simulink model "Project4_MODEL_FINAL"  (R2024b)
settings: Solver=ode45  StartTime=0.0  StopTime=600  RelTol=1e-3
values from neighbouring files (symbols this model uses):
  x_center = [x1 x2_adjusted transition_x x3_adjusted x4]    [Project4_FINAL_Script.m]
  y_center = [y1 y2_adjusted transition_y y3_adjusted y4]    [Project4_FINAL_Script.m]
undefined symbols (not defined in the file or in its folder): BattData, carData, motorData
libraries: slpidlib x1
settings Model: Creator=saman  LastModifiedBy=gabes
settings RTWCC: GPUComputeCapability=3.5

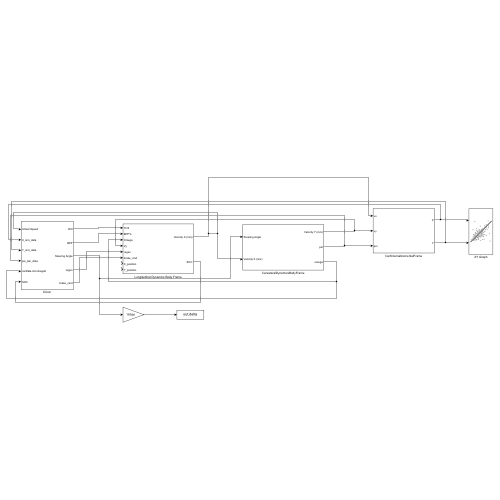
[thumbnail: Simulink's stored preview of the top-level diagram]
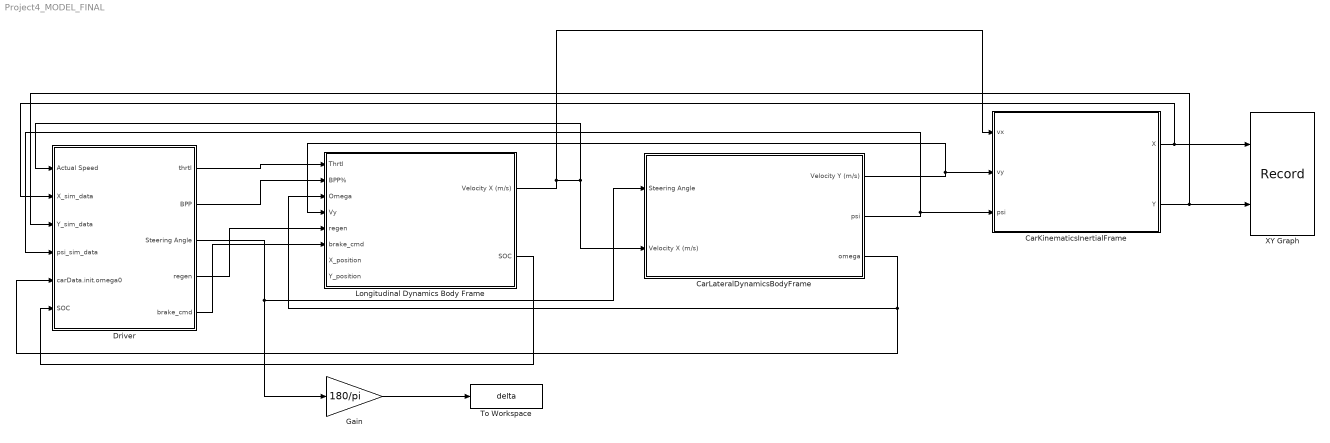
== system Project4_MODEL_FINAL ==
  CarKinematicsInertialFrame : Subsystem
  CarLateralDynamicsBodyFrame : Subsystem
  "Driver " : Subsystem
  Gain : Gain  Gain=180/pi
  Longitudinal Dynamics Body Frame : Subsystem
  To Workspace : ToWorkspace  VariableName=delta  SaveFormat=Timeseries  SampleTime=-1
  XY Graph : Record  FileSettingsInternal="{\"entries\":[{\"content\":{\"excelSettings\":{\"content\":{},\"type\":\"Streamout.ExcelSettings\"}},\"type\":\"Streamout.FileSettingStorage\",\"uuid\":\"\"}],\"packageUris\":[\"http:\\/\\/schema.mathworks.com\\/mf0\\/streamout_blocks\\/R2020a\"],\"version\":\"1.0\"}"  Layout=[1 1]  SignalsInternal="{\"entries\":[{\"content\":{\"signals\":[{\"content\":{\"blockPath\":[],\"dimensions\":[1],\"domain\":\"\",\"lineColor\":\"#a2142f\",\"plots\":[ 1 ],\"port\":1,\"sid\":[\"\"],\"signalID\":1,\"signalName\":\"CarKinematicsInertialFrame:1\"},\"type\":\"RecordBlkView.Signal\",\"uuid\":\"\"},{\"content\":{\"blockPath\":[],\"dimensions\":[1],\"domain\":\"\",\"lineColor\":\"#139fff\",\"plots\":[ 1 ],\"port\":2,\"sid\":[\"\"],\"signalID\":2,\"signalName\":\"CarKinematicsInertialFrame:2\"},\"type\":\"RecordBlkView.Signal\",\"uuid\":\"\"}]},\"type\":\"RecordBlkView.InputSignals\",\"uuid\":\"\"}],\"packageUris\":[\"http:\\/\\/schema.mathworks.com\\/mf0\\/streamout_blocks\\/R2020a\"],\"version\":\"1.0\"}"  VisualizationBindings="{\"xyplotplugin\":{\"info\":[{\"series\":[{\"bindingParametersList\":[{\"parameter\":\"X-Axis\",\"signalID\":1,\"signalName\":\"CarKinematicsInertialFrame:1\"},{\"parameter\":\"Y-Axis\",\"signalID\":2,\"signalName\":\"CarKinematicsInertialFrame:2\"}],\"seriesID\":0}],\"subplotID\":1}]}}"  CompatibilityTag=XY  st=-1
  wires:
  CarLateralDynamicsBodyFrame/2(psi) -> "Driver "/4(psi_sim_data), CarKinematicsInertialFrame/3(psi)
  CarKinematicsInertialFrame/2(Y) -> "Driver "/3(Y_sim_data), XY Graph/2
  CarKinematicsInertialFrame/1(X) -> XY Graph/1, "Driver "/2(X_sim_data)
  CarLateralDynamicsBodyFrame/1(Velocity Y (m/s)) -> Longitudinal Dynamics Body Frame/4(Vy), CarKinematicsInertialFrame/2(vy)
  "Driver "/1(thrtl) -> Longitudinal Dynamics Body Frame/1(Thrtl)
  "Driver "/2(BPP) -> Longitudinal Dynamics Body Frame/2(BPP%)
  Longitudinal Dynamics Body Frame/1(Velocity X (m/s)) -> CarKinematicsInertialFrame/1(vx), "Driver "/1(Actual Speed), CarLateralDynamicsBodyFrame/2(Velocity X (m/s))
  Longitudinal Dynamics Body Frame/2(SOC) -> "Driver "/6(SOC)
  CarLateralDynamicsBodyFrame/3(omega) -> Longitudinal Dynamics Body Frame/3(Omega), "Driver "/5(carData.init.omega0)
  "Driver "/3(Steering Angle) -> Gain/1, CarLateralDynamicsBodyFrame/1(Steering Angle)
  Gain/1 -> To Workspace/1
  "Driver "/4(regen) -> Longitudinal Dynamics Body Frame/5(regen)
  "Driver "/5(brake_cmd) -> Longitudinal Dynamics Body Frame/6(brake_cmd)

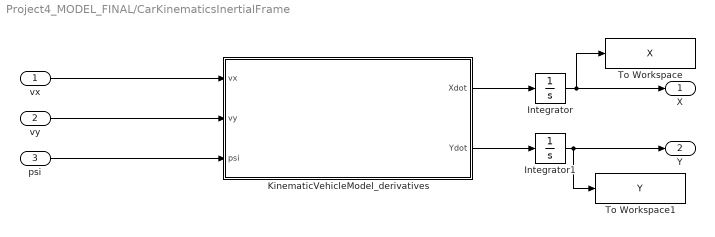
== system Project4_MODEL_FINAL/CarKinematicsInertialFrame ==
  vx : Inport
  vy : Inport  Port=2
  psi : Inport  Port=3
  Integrator : Integrator  InitialCondition=carData.init.x0
  Integrator1 : Integrator  InitialCondition=carData.init.y0
  KinematicVehicleModel_derivatives : MATLAB Function  TreatAsAtomicUnit=on  mask{obj=carData}
      mask prompts: obj "obj structure"
  To Workspace : ToWorkspace  VariableName=X  SaveFormat=Timeseries  SampleTime=-1
  To Workspace1 : ToWorkspace  VariableName=Y  SaveFormat=Timeseries  SampleTime=-1
  X : Outport
  Y : Outport  Port=2
  wires:
  KinematicVehicleModel_derivatives/1(Xdot) -> Integrator/1
  KinematicVehicleModel_derivatives/2(Ydot) -> Integrator1/1
  Integrator/1 -> To Workspace/1, X/1
  Integrator1/1 -> To Workspace1/1, Y/1
  vx/1 -> KinematicVehicleModel_derivatives/1(vx)
  vy/1 -> KinematicVehicleModel_derivatives/2(vy)
  psi/1 -> KinematicVehicleModel_derivatives/3(psi)

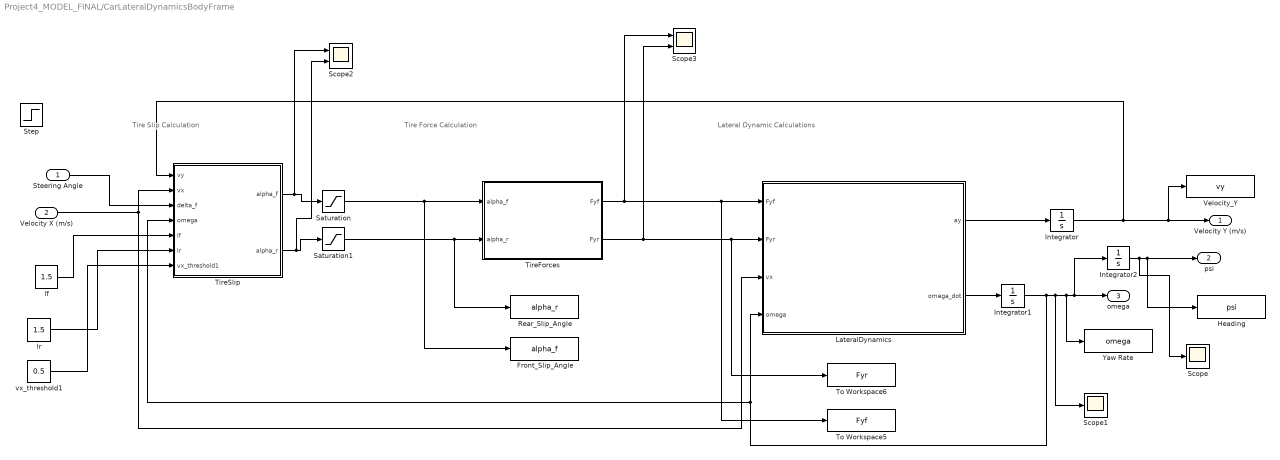
== system Project4_MODEL_FINAL/CarLateralDynamicsBodyFrame ==
  note: Tire Slip Calculation
  note: Tire Force Calculation
  note: Lateral Dynamic Calculations
  Steering Angle : Inport
  Velocity X (m/s) : Inport  Port=2
  Front_Slip_Angle : ToWorkspace  VariableName=alpha_f  SaveFormat=Timeseries  SampleTime=-1
  Heading : ToWorkspace  VariableName=psi  SaveFormat=Timeseries  SampleTime=-1
  Integrator : Integrator  InitialCondition=carData.init.vy0
  Integrator1 : Integrator  InitialCondition=carData.init.omega0
  Integrator2 : Integrator  InitialCondition=carData.init.psi0
  LateralDynamics : MATLAB Function  TreatAsAtomicUnit=on  mask{obj=carData}
      mask prompts: obj "obj structure"
  Rear_Slip_Angle : ToWorkspace  VariableName=alpha_r  SaveFormat=Timeseries  SampleTime=-1
  Saturation : Saturate  UpperLimit=carData.maxAlpha  LowerLimit=-carData.maxAlpha
  Saturation1 : Saturate  UpperLimit=carData.maxAlpha  LowerLimit=-carData.maxAlpha
  Scope : Scope
  Scope1 : Scope
  Scope2 : Scope  NumInputPorts=2
  Scope3 : Scope  NumInputPorts=2
  Step : Step  Time=180  SampleTime=10
  TireForces : MATLAB Function  TreatAsAtomicUnit=on  mask{obj=carData}
      mask prompts: obj "obj structure"
  TireSlip : MATLAB Function  TreatAsAtomicUnit=on  mask{obj=carData}
      mask prompts: obj "obj structure"
  To Workspace5 : ToWorkspace  VariableName=Fyf  SaveFormat=Timeseries  SampleTime=-1
  To Workspace6 : ToWorkspace  VariableName=Fyr  SaveFormat=Timeseries  SampleTime=-1
  Velocity_Y : ToWorkspace  VariableName=vy  SaveFormat=Timeseries  SampleTime=-1
  Yaw Rate : ToWorkspace  VariableName=omega  SaveFormat=Timeseries  SampleTime=-1
  lf : Constant  Value=1.5
  lr : Constant  Value=1.5
  vx_threshold1 : Constant  Value=0.5
  Velocity Y (m/s) : Outport
  psi : Outport  Port=2
  omega : Outport  Port=3
  wires:
  LateralDynamics/1(ay) -> Integrator/1
  Integrator/1 -> Velocity Y (m/s)/1, Velocity_Y/1, TireSlip/1(vy)
  LateralDynamics/2(omega_dot) -> Integrator1/1
  Integrator1/1 -> Scope1/1, Integrator2/1, omega/1, Yaw Rate/1, LateralDynamics/4(omega), TireSlip/4(omega)
  TireSlip/1(alpha_f) -> Scope2/1, Saturation/1
  TireSlip/2(alpha_r) -> Scope2/2, Saturation1/1
  TireForces/2(Fyr) -> Scope3/2, LateralDynamics/2(Fyr), To Workspace6/1
  Saturation/1 -> TireForces/1(alpha_f), Front_Slip_Angle/1
  Saturation1/1 -> TireForces/2(alpha_r), Rear_Slip_Angle/1
  Velocity X (m/s)/1 -> TireSlip/2(vx), LateralDynamics/3(vx)
  Integrator2/1 -> Scope/1, Heading/1, psi/1
  vx_threshold1/1 -> TireSlip/7(vx_threshold1)
  lf/1 -> TireSlip/5(lf)
  lr/1 -> TireSlip/6(lr)
  TireForces/1(Fyf) -> Scope3/1, To Workspace5/1, LateralDynamics/1(Fyf)
  Steering Angle/1 -> TireSlip/3(delta_f)

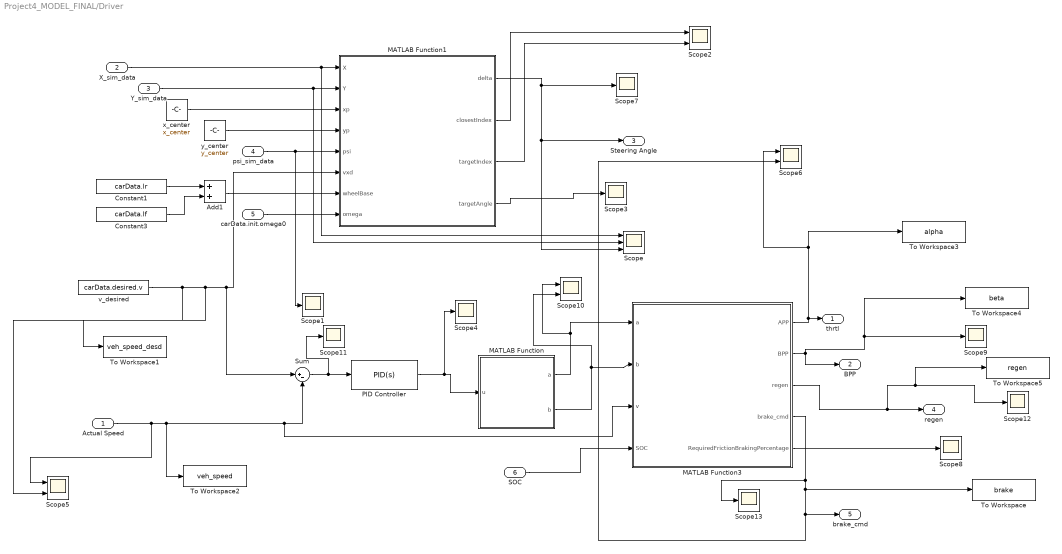
== system Project4_MODEL_FINAL/Driver  ==
  Actual Speed : Inport
  X_sim_data : Inport  Port=2
  Y_sim_data : Inport  Port=3
  psi_sim_data : Inport  Port=4
  carData.init.omega0 : Inport  Port=5
  SOC : Inport  Port=6
  Add1 : Sum
  Constant1 : Constant  Value=carData.lr
  Constant3 : Constant  Value=carData.lf
  MATLAB Function : MATLAB Function  TreatAsAtomicUnit=on
  MATLAB Function1 : MATLAB Function  TreatAsAtomicUnit=on
  MATLAB Function3 : MATLAB Function  TreatAsAtomicUnit=on
  PID Controller : slpidlib/PID Controller  Controller=PID  Form=Parallel  TimeDomain=Continuous-time  UseExternalTs=off  SampleTime=-1  IntegratorMethod=Forward Euler  FilterMethod=Forward Euler  ControllerParametersSource=internal  P=1  I=.2  UseKiTs=off  D=.1  UseExternalDerivativeSource=off  N=50  UseFilter=on  TunerSelectOption=Transfer Function Based (PID Tuner App)  InitialConditionSource=internal  InitialConditionForIntegrator=0  InitialConditionForFilter=0  DifferentiatorICPrevScaledInput=0  ExternalReset=none  TrackingMode=off  Kt=1  LimitOutput=on  SatLimitsSource=internal  UpperSaturationLimit=1  LowerSaturationLimit=-1  LinearizeAsGain=off  AntiWindupMode=clamping  Kb=1  LimitIntegrator=off  UpperIntegratorSaturationLimit=inf  LowerIntegratorSaturationLimit=-inf  POutMin=[]  POutMax=[]  IOutMin=[]  IOutMax=[]  DOutMin=[]  DOutMax=[]  NOutMin=[]  NOutMax=[]  SumOutMin=[]  SumOutMax=[]  SaturationOutMin=[]  SaturationOutMax=[]  PParamMin=[]  PParamMax=[]  IParamMin=[]  IParamMax=[]  DParamMin=[]  DParamMax=[]  NParamMin=[]  NParamMax=[]  KbParamMin=[]  KbParamMax=[]  KtParamMin=[]  KtParamMax=[]  KbOutMin=[]  KbOutMax=[]  KtOutMin=[]  KtOutMax=[]  IntegratorOutMin=[]  IntegratorOutMax=[]  FilterOutMin=[]  FilterOutMax=[]  SumI1OutMin=[]  SumI1OutMax=[]  SumI2OutMin=[]  SumI2OutMax=[]  SumI3OutMin=[]  SumI3OutMax=[]  SumI4OutMin=[]  SumI4OutMax=[]  SumDOutMin=[]  SumDOutMax=[]  DifferentiatorOutMin=[]  DifferentiatorOutMax=[]  FilterDiffOutCoefMin=[]  FilterDiffOutCoefMax=[]  ReciprocalOutMin=[]  ReciprocalOutMax=[]  SumDenOutMin=[]  SumDenOutMax=[]  SumNumOutMin=[]  SumNumOutMax=[]  DivideOutMin=[]  DivideOutMax=[]  UdiffTsProdOutMin=[]  UdiffTsProdOutMax=[]  NTsProdOutMin=[]  NTsProdOutMax=[]  UintegralTsProdOutMin=[]  UintegralTsProdOutMax=[]  UngainTsProdOutMin=[]  UngainTsProdOutMax=[]  ClampingZeroOutDataTypeStr=Inherit: Inherit via back propagation  ClampingZeroOutMin=[]  ClampingZeroOutMax=[]  FilterDenConstantOutDataTypeStr=Inherit: Inherit via back propagation  FilterDenConstantOutMin=[]  FilterDenConstantOutMax=[]  PCopyOutDataTypeStr=Inherit: Inherit via back propagation  PCopyOutMin=[]  PCopyOutMax=[]  NCopyOutDataTypeStr=Inherit: Inherit via back propagation  NCopyOutMin=[]  NCopyOutMax=[]  IntegratorContinuousStateAttributes=''  IntegratorStateMustResolveToSignalObject=off  IntegratorRTWStateStorageClass=Auto  FilterContinuousStateAttributes=''  FilterStateMustResolveToSignalObject=off  FilterRTWStateStorageClass=Auto  ParallelPVariant=InternalParameters  IdealPVariant=Disabled  IVariant=InternalParameters  DVariant=InternalParameters  IntegratorVariant=Continuous  SatVariant=Enabled  AWVariant=ContClampingParallel  PCopyVariant=Disabled  TRVariant=Disabled  FdbkBlocksVariant=Forward  IdealPFdbkVariant=Disabled  SatFdbkVariant=Disabled  DerivativeFilterVariant=ContFilter  NVariant=InternalParameters  NCopyVariant=Disabled  FilterICVariant=InternalICsFilter  IntegratorICVariant=InternalICs  ExternalResetVariant=Disabled  TRSumVariant=Passthrough  SumFdbkVariant=Disabled  SumVariant=Sum_PID  TsampFilterVariant=InternalTs  TsampNgainVariant=Passthrough  TsampIntegralVariant=Disabled_SignalSpec  ExternalSaturationOutDataTypeStr=Inherit: Same as second input  DerivativeSourceVariant=ErrorSignal  PreIntVariant=InternalPreInt
  Scope : Scope  NumInputPorts=3
  Scope{1,3..4,7..9,11..13} (9 alike) : Scope
  Scope{2,5..6,10} (4 alike) : Scope  NumInputPorts=2
  Sum : Sum  Inputs=|+-
  To Workspace : ToWorkspace  VariableName=brake  SaveFormat=Timeseries  SampleTime=-1
  To Workspace1 : ToWorkspace  VariableName=veh_speed_desd  SaveFormat=Timeseries  SampleTime=-1
  To Workspace2 : ToWorkspace  VariableName=veh_speed  SaveFormat=Timeseries  SampleTime=-1
  To Workspace3 : ToWorkspace  VariableName=alpha  SaveFormat=Timeseries  SampleTime=-1
  To Workspace4 : ToWorkspace  VariableName=beta  SaveFormat=Timeseries  SampleTime=-1
  To Workspace5 : ToWorkspace  VariableName=regen  SaveFormat=Timeseries  SampleTime=-1
  v_desired : Constant  Value=carData.desired.v
  x_center : Constant  Value=x_center  VectorParams1D=off
  y_center : Constant  Value=y_center  VectorParams1D=off
  thrtl : Outport
  BPP : Outport  Port=2
  Steering Angle : Outport  Port=3
  regen : Outport  Port=4
  brake_cmd : Outport  Port=5
  wires:
  v_desired/1 -> To Workspace1/1, Scope5/2, Sum/1, MATLAB Function1/6(vxd)
  Actual Speed/1 -> Scope5/1, To Workspace2/1, MATLAB Function3/3(v), Sum/2
  Sum/1 -> Scope11/1, PID Controller/1
  PID Controller/1 -> Scope4/1, MATLAB Function/1(u)
  carData.init.omega0/1 -> MATLAB Function1/8(omega)
  y_center/1 -> MATLAB Function1/4(yp)
  psi_sim_data/1 -> Scope1/1, MATLAB Function1/5(psi)
  X_sim_data/1 -> Scope/1, MATLAB Function1/1(X)
  x_center/1 -> MATLAB Function1/3(xp)
  MATLAB Function1/1(delta) -> Steering Angle/1, Scope/3, Scope7/1
  Y_sim_data/1 -> Scope/2, MATLAB Function1/2(Y)
  Constant3/1 -> Add1/2
  Constant1/1 -> Add1/1
  Add1/1 -> MATLAB Function1/7(wheelBase)
  MATLAB Function/1(a) -> Scope10/1, MATLAB Function3/1(a)
  MATLAB Function/2(b) -> Scope10/2, MATLAB Function3/2(b)
  SOC/1 -> MATLAB Function3/4(SOC)
  MATLAB Function3/2(BPP) -> BPP/1, Scope9/1, To Workspace4/1
  MATLAB Function3/1(APP) -> Scope6/1, To Workspace3/1, thrtl/1
  MATLAB Function1/2(closestIndex) -> Scope2/1
  MATLAB Function1/3(targetIndex) -> Scope2/2
  MATLAB Function1/4(targetAngle) -> Scope3/1
  MATLAB Function3/4(brake_cmd) -> Scope13/1, brake_cmd/1, Scope6/2, To Workspace/1
  MATLAB Function3/5(RequiredFrictionBrakingPercentage) -> Scope8/1
  MATLAB Function3/3(regen) -> regen/1, To Workspace5/1, Scope12/1

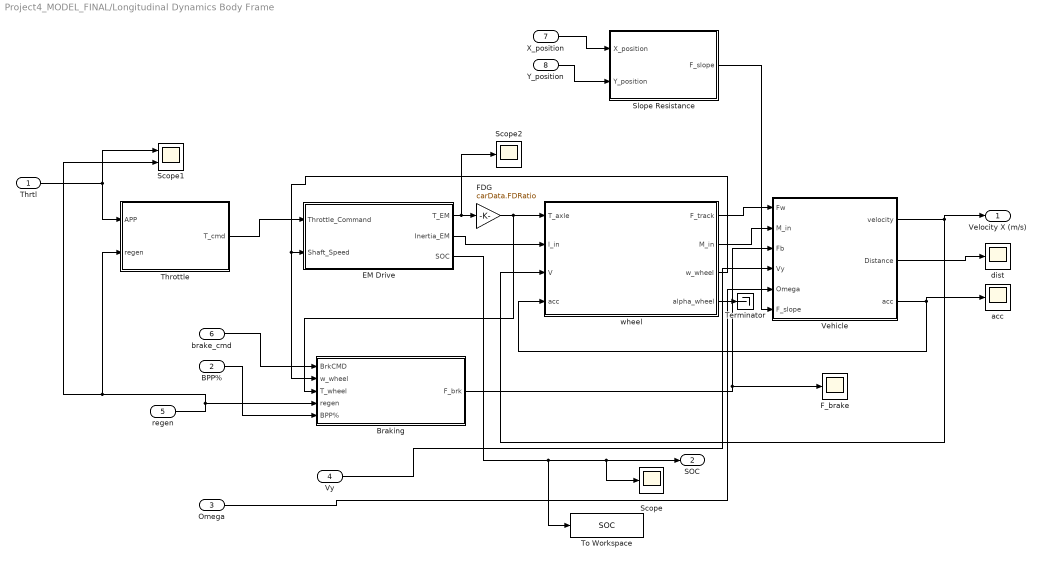
== system Project4_MODEL_FINAL/Longitudinal Dynamics Body Frame ==
  Thrtl : Inport
  BPP% : Inport  Port=2
  Omega : Inport  Port=3
  Vy : Inport  Port=4
  regen : Inport  Port=5
  brake_cmd : Inport  Port=6
  X_position : Inport  Port=7
  Y_position : Inport  Port=8
  Braking : Subsystem
  EM Drive : Subsystem
  FDG : Gain  Gain=carData.FDRatio
  F_brake : Scope
  Scope : Scope
  Scope1 : Scope  NumInputPorts=2
  Scope2 : Scope
  "Slope Resistance " : Subsystem
  Terminator : Terminator
  Throttle : Subsystem
  To Workspace : ToWorkspace  VariableName=SOC  SaveFormat=Timeseries  SampleTime=-1
  Vehicle : Subsystem
  acc : Scope
  dist : Scope
  "wheel " : Subsystem
  Velocity X (m/s) : Outport
  SOC : Outport  Port=2
  wires:
  "wheel "/3(w_wheel) -> Braking/2("w_wheel "), EM Drive/2(Shaft_Speed)
  Vehicle/3(acc) -> acc/1, "wheel "/4(acc)
  Braking/1("F_brk ") -> Vehicle/3("Fb "), F_brake/1
  "wheel "/2(M_in) -> Vehicle/2("M_in ")
  Vehicle/1("velocity ") -> Velocity X (m/s)/1, "wheel "/3(V)
  "wheel "/1(F_track) -> Vehicle/1("Fw ")
  EM Drive/3(SOC) -> To Workspace/1, Scope/1, SOC/1
  FDG/1 -> Braking/3(T_wheel), "wheel "/1(T_axle)
  EM Drive/2(Inertia_EM) -> "wheel "/2(I_in)
  Vehicle/2("Distance ") -> dist/1
  "wheel "/4(alpha_wheel) -> Terminator/1
  EM Drive/1(T_EM) -> Scope2/1, FDG/1
  BPP%/1 -> Braking/5(BPP%)
  Vy/1 -> Vehicle/4(Vy)
  Omega/1 -> Vehicle/5(Omega)
  regen/1 -> Scope1/2, Throttle/2(regen), Braking/4(regen)
  Thrtl/1 -> Scope1/1, Throttle/1(APP)
  Throttle/1(T_cmd) -> EM Drive/1(Throttle_Command)
  brake_cmd/1 -> Braking/1("BrkCMD ")
  X_position/1 -> "Slope Resistance "/1(X_position)
  Y_position/1 -> "Slope Resistance "/2(Y_position)
  "Slope Resistance "/1(F_slope) -> Vehicle/6(F_slope)

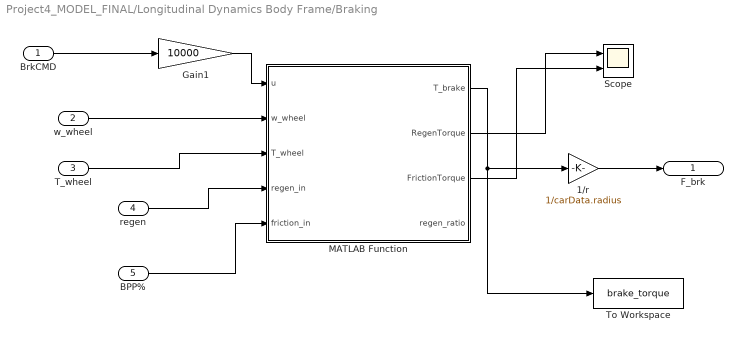
== system Project4_MODEL_FINAL/Longitudinal Dynamics Body Frame/Braking ==
  "BrkCMD " : Inport
  "w_wheel " : Inport  Port=2
  T_wheel : Inport  Port=3
  regen : Inport  Port=4
  BPP% : Inport  Port=5
  1/r : Gain  Gain=1/carData.radius
  Gain1 : Gain  Gain=10000
  MATLAB Function : MATLAB Function  TreatAsAtomicUnit=on
  Scope : Scope  NumInputPorts=2
  To Workspace : ToWorkspace  VariableName=brake_torque  SaveFormat=Timeseries  SampleTime=-1
  "F_brk " : Outport  VectorParamsAs1DForOutWhenUnconnected=off
  wires:
  "BrkCMD "/1 -> Gain1/1
  Gain1/1 -> MATLAB Function/1(u)
  MATLAB Function/1(T_brake) -> To Workspace/1, 1/r/1
  "w_wheel "/1 -> MATLAB Function/2(w_wheel)
  T_wheel/1 -> MATLAB Function/3(T_wheel)
  1/r/1 -> "F_brk "/1
  regen/1 -> MATLAB Function/4(regen_in)
  BPP%/1 -> MATLAB Function/5(friction_in)
  MATLAB Function/2(RegenTorque) -> Scope/1
  MATLAB Function/3(FrictionTorque) -> Scope/2

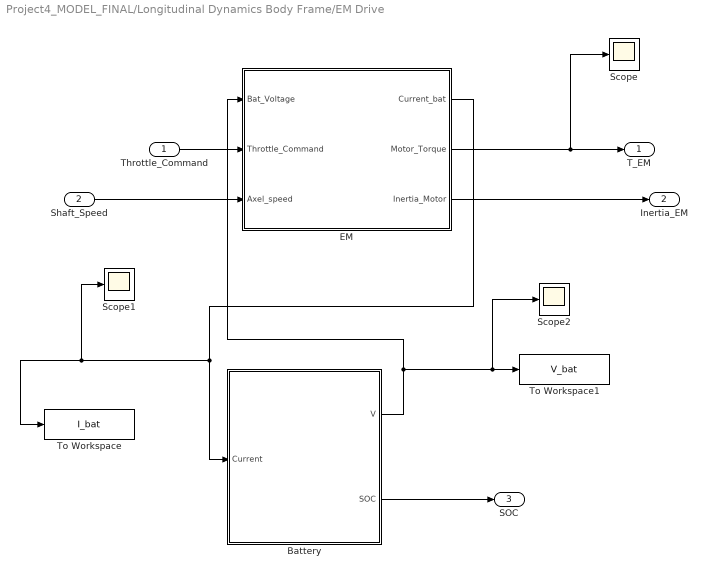
== system Project4_MODEL_FINAL/Longitudinal Dynamics Body Frame/EM Drive ==
  Throttle_Command : Inport
  Shaft_Speed : Inport  Port=2
  Battery : Subsystem
  EM : Subsystem
  Scope : Scope
  Scope1 : Scope
  Scope2 : Scope
  To Workspace : ToWorkspace  VariableName=I_bat  SaveFormat=Timeseries  SampleTime=.5
  To Workspace1 : ToWorkspace  VariableName=V_bat  SaveFormat=Timeseries  SampleTime=.5
  T_EM : Outport
  Inertia_EM : Outport  Port=2
  SOC : Outport  Port=3
  wires:
  EM/1(Current_bat) -> Scope1/1, To Workspace/1, Battery/1(Current)
  Throttle_Command/1 -> EM/2(Throttle_Command)
  Shaft_Speed/1 -> EM/3(Axel_speed)
  EM/2(Motor_Torque) -> Scope/1, T_EM/1
  EM/3(Inertia_Motor) -> Inertia_EM/1
  Battery/1(V) -> Scope2/1, To Workspace1/1, EM/1(Bat_Voltage)
  Battery/2(SOC) -> SOC/1

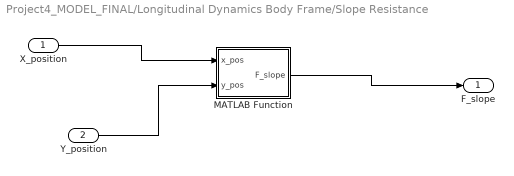
== system Project4_MODEL_FINAL/Longitudinal Dynamics Body Frame/Slope Resistance  ==
  X_position : Inport
  Y_position : Inport  Port=2
  MATLAB Function : MATLAB Function  TreatAsAtomicUnit=on
  F_slope : Outport
  wires:
  X_position/1 -> MATLAB Function/1(x_pos)
  Y_position/1 -> MATLAB Function/2(y_pos)
  MATLAB Function/1(F_slope) -> F_slope/1

== system Project4_MODEL_FINAL/Longitudinal Dynamics Body Frame/Throttle ==
  APP : Inport
  regen : Inport  Port=2
  MATLAB Function : MATLAB Function  TreatAsAtomicUnit=on
  T_cmd : Outport
  wires:
  MATLAB Function/1(T_cmd) -> T_cmd/1
  APP/1 -> MATLAB Function/1(APP)
  regen/1 -> MATLAB Function/2(regen)

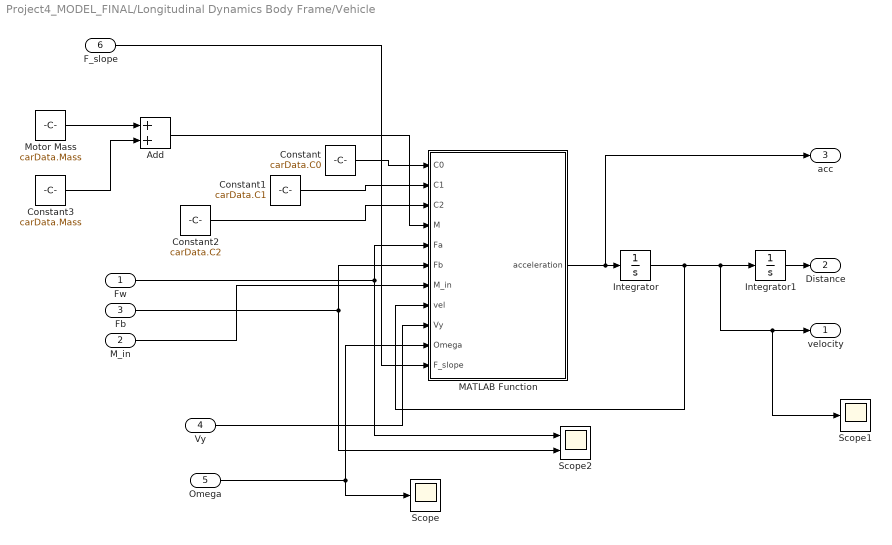
== system Project4_MODEL_FINAL/Longitudinal Dynamics Body Frame/Vehicle ==
  "Fw " : Inport
  "M_in " : Inport  Port=2
  "Fb " : Inport  Port=3
  Vy : Inport  Port=4
  Omega : Inport  Port=5
  F_slope : Inport  Port=6
  Add : Sum
  Constant : Constant  Value=carData.C0
  Constant1 : Constant  Value=carData.C1
  Constant2 : Constant  Value=carData.C2
  Constant3 : Constant  Value=carData.Mass
  Integrator : Integrator  LimitOutput=on  LowerSaturationLimit=0
  Integrator1 : Integrator
  MATLAB Function : MATLAB Function  TreatAsAtomicUnit=on
  Motor Mass : Constant  Value=carData.Mass
  Scope : Scope
  Scope1 : Scope
  Scope2 : Scope  NumInputPorts=2
  "velocity " : Outport  VectorParamsAs1DForOutWhenUnconnected=off
  "Distance " : Outport  Port=2  VectorParamsAs1DForOutWhenUnconnected=off
  acc : Outport  Port=3
  wires:
  Constant1/1 -> MATLAB Function/2(C1)
  Constant/1 -> MATLAB Function/1(C0)
  MATLAB Function/1(acceleration) -> acc/1, Integrator/1
  Constant2/1 -> MATLAB Function/3(C2)
  Constant3/1 -> Add/2
  "Fw "/1 -> Scope2/1, MATLAB Function/5(Fa)
  "Fb "/1 -> Scope2/2, MATLAB Function/6(Fb)
  Integrator/1 -> MATLAB Function/8(vel), Scope1/1, "velocity "/1, Integrator1/1
  Integrator1/1 -> "Distance "/1
  "M_in "/1 -> MATLAB Function/7(M_in)
  Motor Mass/1 -> Add/1
  Add/1 -> MATLAB Function/4(M)
  Vy/1 -> MATLAB Function/9(Vy)
  Omega/1 -> Scope/1, MATLAB Function/10(Omega)
  F_slope/1 -> MATLAB Function/11(F_slope)

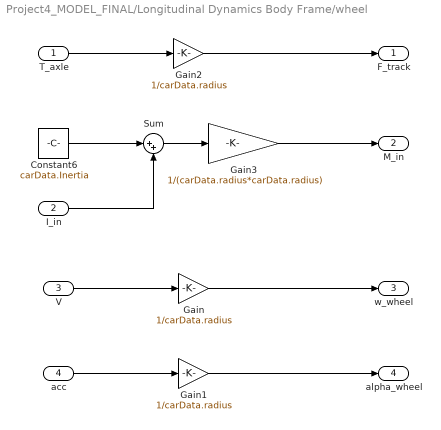
== system Project4_MODEL_FINAL/Longitudinal Dynamics Body Frame/wheel  ==
  T_axle : Inport
  I_in : Inport  Port=2
  V : Inport  Port=3
  acc : Inport  Port=4
  Constant6 : Constant  Value=carData.Inertia
  Gain : Gain  Gain=1/carData.radius
  Gain1 : Gain  Gain=1/carData.radius
  Gain2 : Gain  Gain=1/carData.radius
  Gain3 : Gain  Gain=1/(carData.radius*carData.radius)
  Sum : Sum  Inputs=|++
  F_track : Outport
  M_in : Outport  Port=2
  w_wheel : Outport  Port=3
  alpha_wheel : Outport  Port=4
  wires:
  Gain/1 -> w_wheel/1
  V/1 -> Gain/1
  acc/1 -> Gain1/1
  Gain1/1 -> alpha_wheel/1
  T_axle/1 -> Gain2/1
  Gain2/1 -> F_track/1
  Gain3/1 -> M_in/1
  Constant6/1 -> Sum/1
  I_in/1 -> Sum/2
  Sum/1 -> Gain3/1

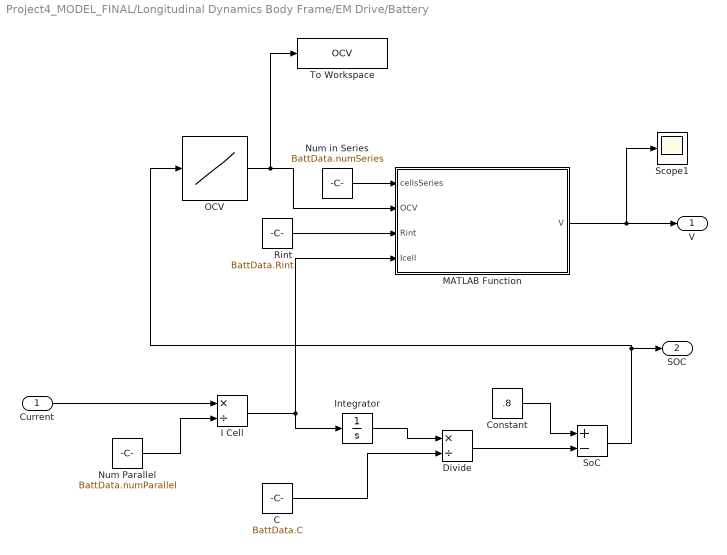
== system Project4_MODEL_FINAL/Longitudinal Dynamics Body Frame/EM Drive/Battery ==
  Current : Inport
  C : Constant  Value=BattData.C
  Constant : Constant  Value=.8
  Divide : Product  Inputs=*/
  I Cell : Product  Inputs=*/
  Integrator : Integrator
  MATLAB Function : MATLAB Function  TreatAsAtomicUnit=on
  Num Parallel : Constant  Value=BattData.numParallel
  Num in Series : Constant  Value=BattData.numSeries
  OCV : Lookup_n-D  NumberOfTableDimensions=1  BreakpointsForDimension1=BattData.SOC  BreakpointsForDimension2=[1:3]  Table=BattData.OCV  InternalRulePriority=Speed  RndMeth=Simplest
  Rint : Constant  Value=BattData.Rint
  Scope1 : Scope
  SoC : Sum  Inputs=+-
  To Workspace : ToWorkspace  VariableName=OCV  SaveFormat=Timeseries  SampleTime=.5
  V : Outport
  SOC : Outport  Port=2
  wires:
  Num Parallel/1 -> I Cell/2
  I Cell/1 -> Integrator/1, MATLAB Function/4(Icell)
  C/1 -> Divide/2
  Integrator/1 -> Divide/1
  Divide/1 -> SoC/2
  SoC/1 -> SOC/1, OCV/1
  MATLAB Function/1(V) -> Scope1/1, V/1
  OCV/1 -> To Workspace/1, MATLAB Function/2(OCV)
  Rint/1 -> MATLAB Function/3(Rint)
  Num in Series/1 -> MATLAB Function/1(cellsSeries)
  Constant/1 -> SoC/1
  Current/1 -> I Cell/1

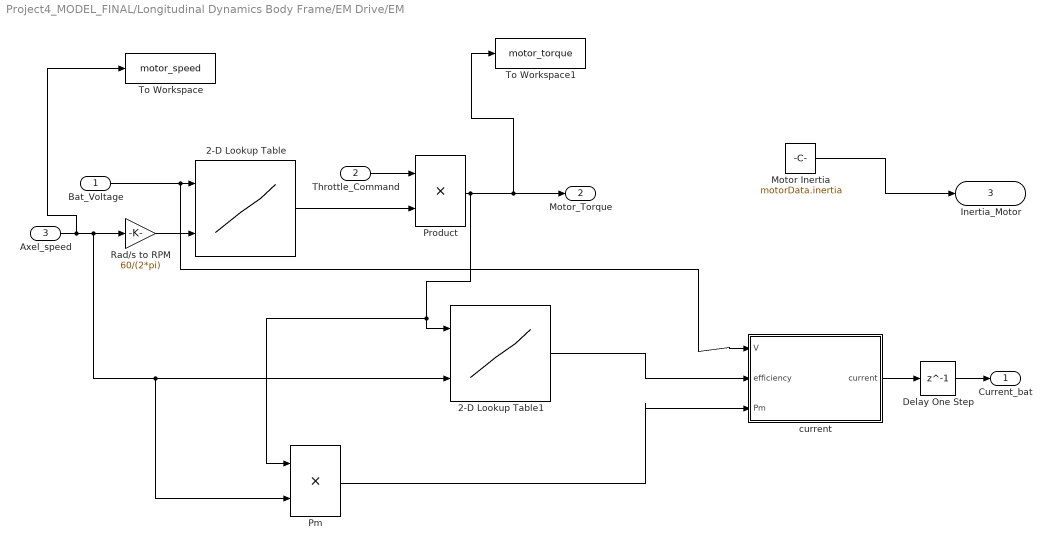
== system Project4_MODEL_FINAL/Longitudinal Dynamics Body Frame/EM Drive/EM ==
  Bat_Voltage : Inport
  Throttle_Command : Inport  Port=2
  Axel_speed : Inport  Port=3
  2-D Lookup Table : Lookup_n-D  BreakpointsForDimension1=motorData.vbus  BreakpointsForDimension2=motorData.rpm  Table=motorData.maxtorque  InternalRulePriority=Speed  RndMeth=Simplest
      settings: InputPortMap=u0,u1
  2-D Lookup Table1 : Lookup_n-D  BreakpointsForDimension1=motorData.eta_torque  BreakpointsForDimension2=motorData.eta_speed  Table=motorData.eta_val  InternalRulePriority=Speed  RndMeth=Simplest
      settings: InputPortMap=u0,u1
  Delay One Step : Delay  DelayLength=1  SampleTime=.5
  Motor Inertia : Constant  Value=motorData.inertia
  Pm : Product
  Product : Product
  Rad/s to RPM : Gain  Gain=60/(2*pi)
  To Workspace : ToWorkspace  VariableName=motor_speed  SaveFormat=Timeseries  SampleTime=.5
  To Workspace1 : ToWorkspace  VariableName=motor_torque  SaveFormat=Timeseries  SampleTime=.5
  current : MATLAB Function  TreatAsAtomicUnit=on
  Current_bat : Outport
  Motor_Torque : Outport  Port=2
  Inertia_Motor : Outport  Port=3
  wires:
  Axel_speed/1 -> To Workspace/1, Rad/s to RPM/1, 2-D Lookup Table1/2, Pm/2
  Bat_Voltage/1 -> current/1(V), 2-D Lookup Table/1
  2-D Lookup Table/1 -> Product/2
  Throttle_Command/1 -> Product/1
  Product/1 -> Pm/1, 2-D Lookup Table1/1, To Workspace1/1, Motor_Torque/1
  Pm/1 -> current/3(Pm)
  2-D Lookup Table1/1 -> current/2(efficiency)
  Motor Inertia/1 -> Inertia_Motor/1
  current/1(current) -> Delay One Step/1
  Rad/s to RPM/1 -> 2-D Lookup Table/2
  Delay One Step/1 -> Current_bat/1

== matlab function Project4_MODEL_FINAL/CarLateralDynamicsBodyFrame/TireForces ==
  data: alpha_f input; alpha_r input; Fyf output; obj parameter; Fyr output
function [Fyf, Fyr] = fcn(alpha_f, alpha_r, obj)
    Fyf = max(-obj.fymax, min(obj.fymax, obj.Calphaf * alpha_f));
    Fyr = max(-obj.fymaxR, min(obj.fymaxR, obj.Calphar * alpha_r));
end

== matlab function Project4_MODEL_FINAL/CarLateralDynamicsBodyFrame/TireSlip ==
  data: vy input size=1; vx input; delta_f input size=1; omega input; lf input; alpha_f output; alpha_r output; lr input; vx_threshold1 input
function [alpha_f, alpha_r] = fcn(vy, vx, delta_f, omega, lf, lr, vx_threshold1)

if abs(vx) > vx_threshold1
    %epsilon = 0.01*sign(vx);
    alpha_f = delta_f - (vy + omega * lf) / vx;
    alpha_r = - (vy - omega * lr) / vx;
else
    alpha_f = 0;
    alpha_r = 0;
end


% function [alpha_f, alpha_r] = fcn(vy,  vx, delta_f, omega, obj)
% 
% if abs(vx)> obj.vx_threshold1
%       alpha_f = delta_f - (vy + omega * obj.lf) / vx;
%       alpha_r = - (vy - omega * obj.lr) / vx;
% else
%       alpha_f = 0;
%       alpha_r = 0;
% end
% end
%

== matlab function Project4_MODEL_FINAL/Longitudinal Dynamics Body Frame/Slope Resistance /MATLAB Function ==
  data: x_pos input; F_slope output; y_pos input
function F_slope = computeSlopeForce(x_pos, y_pos)
    %--- Physical Parameters ---
    vehicle_mass = 1000;     % Mass of vehicle in kg
    gravity = 9.81;          % Acceleration due to gravity in m/s^2

    %--- Normalize x position within repeating hill segment (0 to 900 meters) ---
    x_local = mod(x_pos, 900);  % Effective position on repeating hill profile

    %--- Calculate hill gradient using derivative of sigmoid curve ---
    hill_gradient = (10/50) * exp((x_local - 450)/50) / ...
                    ((1 + exp((x_local - 450)/50))^2);

    %--- Determine hill direction based on y position ---
    if y_pos < 200
        elevation_slope = hill_gradient;   % Ascending slope
    else
        elevation_slope = -hill_gradient;  % Descending slope
    end

    %--- Compute gravitational slope force ---
    F_slope = vehicle_mass * gravity * elevation_slope;
end

== matlab function Project4_MODEL_FINAL/Driver /MATLAB Function1 ==
  data: X input; delta output; Y input; xp input; yp input; psi input; vxd input; wheelBase input; omega input; closestIndex output; targetIndex output; targetAngle output
function [delta, closestIndex, targetIndex, targetAngle] = SimplestDriver(X, Y, xp, yp, psi, vxd, wheelBase, omega)
    distances = (xp - X).^2 + (yp - Y).^2;
    [~, closestIndex] = min(distances);
    nPoints = length(xp);

    % Lookahead based on speed
    baseLookahead = 3.0;
    lookaheadFactor = 1.0;
    lookaheadDist = baseLookahead + lookaheadFactor * vxd;
    lookaheadDist = min(50, max(5, lookaheadDist));  % limit bounds

    % Find target waypoint
    targetIndex = closestIndex;
    distanceAhead = 0;
    while distanceAhead < lookaheadDist && targetIndex < nPoints
        targetIndex = targetIndex + 1;
        dx = xp(targetIndex) - X;
        dy = yp(targetIndex) - Y;
        distanceAhead = sqrt(dx^2 + dy^2);
        if targetIndex == nPoints
            break;
        end
    end

    % Compute heading error
    targetX = xp(targetIndex);
    targetY = yp(targetIndex);
    targetAngle = atan2(targetY - Y, targetX - X);
    headingError = atan2(sin(targetAngle - psi), cos(targetAngle - psi));

    % Pure pursuit steering
    headingGain = 2.5;
    targetDistance = max(1.0, sqrt((targetX - X)^2 + (targetY - Y)^2));
    delta_command = atan(2 * wheelBase * sin(headingGain * headingError) / targetDistance);

    % Feedforward correction
    yawDampingGain = 0.05;
    delta = delta_command - yawDampingGain * omega;

    % Clamp
    % maxSteerAngle = 0.5;
    % delta = min(max(delta, -maxSteerAngle), maxSteerAngle);
    % delta= -delta;
end

== matlab function Project4_MODEL_FINAL/Driver /MATLAB Function3 ==
  data: a input; b input; APP output; v input; SOC input; BPP output; regen output; brake_cmd output; RequiredFrictionBrakingPercentage output
% function [APP, BPP, regen] = fcn(a, b, v, SOC)
% if b < 0 % Braking command is zero or negative
%     APP = 0;
%     BPP = abs(b); % Use the magnitude for brake pressure
%     regen = 0.1 * abs(b); % Example: 10% of braking for regen
% else % Acceleration command (b is positive or zero in this case)
%     APP = a;
%     regen = 0;
%     BPP = 0;
% end
% 

function [APP, BPP, regen, brake_cmd, RequiredFrictionBrakingPercentage] = fcn(a, b, v, SOC)
% Inputs:
% a   - acceleration command (positive)
% b   - braking command (negative)
% v   - vehicle speed (m/s)
% SOC - state of charge [0–1]

% Outputs:
% APP  - accelerator pedal position (0–1)
% BPP  - brake pedal pressure (0–1)
% regen - regen command percentage (0–1)
% RequiredFrictionBrakingPercentage - minimum friction braking % needed

% --- Emergency cutoff if battery is dead ---
if SOC <= 0.1
    APP = 0;
    BPP = 0;
    regen = 0;
    brake_cmd = 0;
    RequiredFrictionBrakingPercentage = 1.0;
    return;
end

speed_mph = v;

% --- Determine minimum friction brake requirement based on speed ---
if speed_mph < 5
    RequiredFrictionBrakingPercentage = 1.0;
elseif speed_mph <= 25
    RequiredFrictionBrakingPercentage = 1.0 - ((1.0 - 0.05) / (25 - 5)) * (speed_mph - 5);
else
    RequiredFrictionBrakingPercentage = 0.05;
end

% --- Braking logic ---
if b < 0
    brake_cmd = abs(b);

    % Required friction braking
    BPP = brake_cmd * RequiredFrictionBrakingPercentage;

    % Regen scaling based on SOC
    if SOC >= 0.8
        regenScale = 0.2;
    elseif SOC >= 0.2
        regenScale = 1.0;
    else
        regenScale = 0.5;
    end

    % Regen handles the non-required portion of braking
    regen_fraction = (1 - RequiredFrictionBrakingPercentage) * regenScale;
    regen = brake_cmd * regen_fraction;

    APP = 0;
else
    APP = a;
    BPP = 0;
    regen = 0;
    brake_cmd = 0;
    RequiredFrictionBrakingPercentage = 0;
end
end

== matlab function Project4_MODEL_FINAL/Longitudinal Dynamics Body Frame/Throttle/MATLAB Function ==
  data: APP input; T_cmd output; regen input
function T_cmd = fcn(APP, regen)
    if APP > 0
        T_cmd = APP;
    elseif regen > 0
        T_cmd = -regen;
    else
        T_cmd = 0;
    end
end

== matlab function Project4_MODEL_FINAL/Driver /MATLAB Function ==
  data: u input; a output; b output
function [a,b] = fcn(u)

if u>0
    acc=u;
    brk=0;
elseif u<0
    acc=0;
    brk=u;
else
    acc=0;
    brk=0;
end
a= acc;
b= brk;

== matlab function Project4_MODEL_FINAL/Longitudinal Dynamics Body Frame/Vehicle/MATLAB Function ==
  data: C0 input; acceleration output; C1 input; C2 input; M input; Fa input; Fb input; M_in input; vel input; Vy input; Omega input; F_slope input
function acceleration   = vehicle(C0,C1,C2,M,Fa,Fb,M_in, vel, Vy, Omega, F_slope)

acceleration = (((Fa+Fb - F_slope))-(C0+ C1*vel + C2*(vel)^2))/(M+M_in)+ (Vy*Omega);

== matlab function Project4_MODEL_FINAL/Longitudinal Dynamics Body Frame/EM Drive/EM/current ==
  data: V input; current output; efficiency input; Pm input
function current = fcn(V,efficiency,Pm)

current = (Pm * efficiency^(Pm/(abs(Pm)+0.001))) / max(V, 0.1);

== matlab function Project4_MODEL_FINAL/Longitudinal Dynamics Body Frame/EM Drive/Battery/MATLAB Function ==
  data: cellsSeries input; V output; OCV input; Rint input; Icell input
function V = fcn(cellsSeries,OCV,Rint,Icell)

V = cellsSeries*(OCV-Rint*Icell);

== matlab function Project4_MODEL_FINAL/CarKinematicsInertialFrame/KinematicVehicleModel_derivatives ==
  data: vx input; vy input; psi input size=1; Xdot output; Ydot output
function [Xdot, Ydot] = fcn(vx, vy, psi)
    temp = TF(psi) * [vx;vy]; 
    Xdot = temp(1);
    Ydot = temp(2);
  
end

function y = TF(psi)
    y = [cos(psi), -sin(psi); sin(psi), cos(psi)];
end

== matlab function Project4_MODEL_FINAL/CarLateralDynamicsBodyFrame/LateralDynamics ==
  data: Fyf input; Fyr input size=1; vx input; omega input; ay output; obj parameter; omega_dot output
function [ay, omega_dot] = fcn(Fyf, Fyr, vx, omega, obj)

Fy = Fyf + Fyr;
ay = Fy / obj.Mass - omega * vx;
        
M  = Fyf * obj.lf - Fyr * obj.lr;        
omega_dot = M / obj.Inertia;        

end

== matlab function Project4_MODEL_FINAL/Longitudinal Dynamics Body Frame/Braking/MATLAB Function ==
  data: u input; T_brake output; w_wheel input; T_wheel input; regen_in input; friction_in input; RegenTorque output; FrictionTorque output; regen_ratio output
function [T_brake, RegenTorque, FrictionTorque, regen_ratio] = fcn(u, w_wheel, T_wheel, regen_in, friction_in)
    DesiredBrakingTorqueMagnitude = abs(u); % Magnitude of desired brake torque

    % Calculate the magnitude of friction brake torque required
    epsilon = 1e-6;  % small value to avoid division by zero

    if abs(friction_in) < epsilon
        regen_ratio = 0;
    else
        regen_ratio = regen_in / (regen_in + friction_in);
    end

    % Higher speed: combine friction and regen (simplified)
    RegenTorque = DesiredBrakingTorqueMagnitude * regen_ratio;
    FrictionTorque = DesiredBrakingTorqueMagnitude - RegenTorque;
    TotalBrakeTorqueMagnitude = RegenTorque + FrictionTorque;

    % maxRegenTorque = 0.5 * max(motorData.maxtorque(:));  % say 50% of max torque
    % regenTorque = -regen * maxRegenTorque;

    % Apply braking torque in the opposite direction of motion
    if w_wheel > 1e-3
        T_brake = -TotalBrakeTorqueMagnitude;
    elseif w_wheel < -1e-3
        T_brake = TotalBrakeTorqueMagnitude;
    else % Wheel speed is close to zero
        T_brake = min(abs(T_wheel), TotalBrakeTorqueMagnitude) * sign(w_wheel);
    end
end

% function T_brake = fcn(u, w_wheel, T_wheel)
%     Tb_cap = u;  % Positive brake command
% 
%     if abs(w_wheel) < 1e-3
%         T_brake = min(abs(T_wheel), Tb_cap) * sign(w_wheel);
%     else
%         T_brake = Tb_cap * sign(w_wheel);  % Apply opposite direction of motion
%     end
% end
